simulink model "tutorial39_controller"  (R2025a)
settings: Solver=VariableStepAuto  StartTime=0.0  StopTime=10.0  RelTol=1e-3
InitFcn:
  | Kp_gain = 3;
settings Model: Creator=xing2  LastModifiedBy=xing2

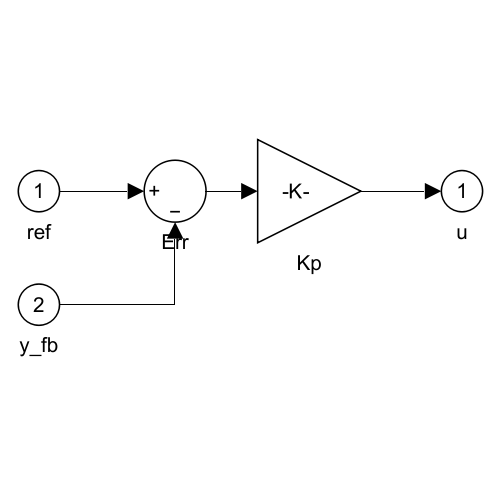
[thumbnail: Simulink's stored preview of the top-level diagram]
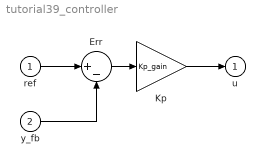
== system tutorial39_controller ==
  ref : Inport
  y_fb : Inport  Port=2
  Err : Sum  Inputs=|+-
  Kp : Gain  Gain=Kp_gain
  u : Outport
  wires:
  y_fb/1 -> Err/2
  ref/1 -> Err/1
  Kp/1 -> u/1
  Err/1 -> Kp/1
